simulink model "mathmeticmodel"  (R2019b)
settings: Solver=VariableStepAuto  StartTime=0.0  StopTime=10  RelTol=1e-3
undefined symbols (not defined in the file): DiscIntNeverNeededParam, eta, Fh, Id0, k, KL, KR, LdRated, LqRated, psi_dh, psi_qh, PsiPMRated, RsRated, TsimFSO, TsimMotor, Ud0, Udh, Uq0, Uqh, we
libraries: simulink x2
settings Model: SimulationMode=accelerator  Creator=Downstream  LastModifiedBy=Downstream
settings DataIOCC: ReturnWorkspaceOutputs=off

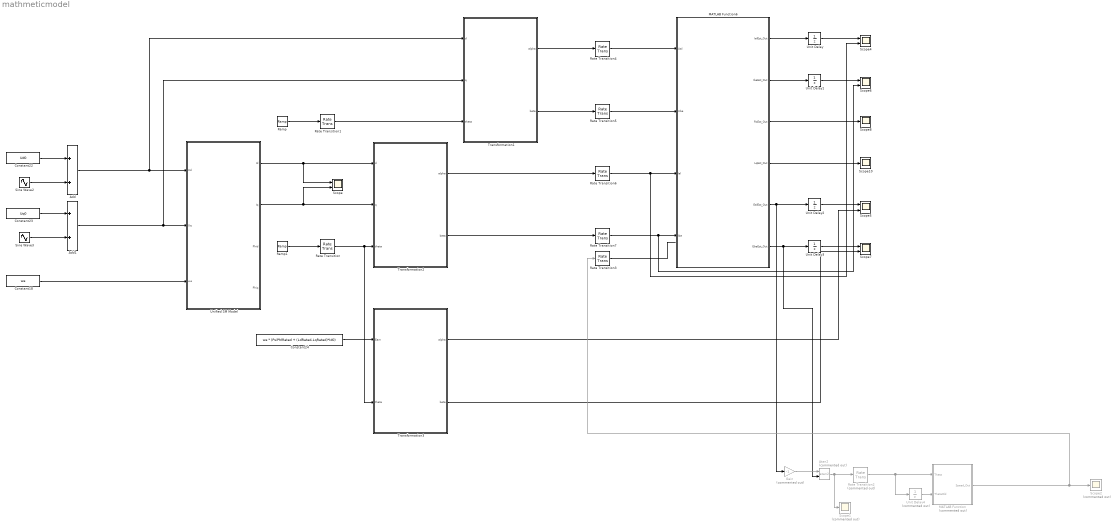
== system mathmeticmodel ==
  Add : Sum
  Add1 : Sum
  Atan2 : Trigonometry  Commented=on  Operator=atan2
  Constant18 : Constant  Value=we  SampleTime=TsimFSO
  Constant22 : Constant  Value=Ud0  SampleTime=TsimFSO
  Constant23 : Constant  Value=Uq0  SampleTime=TsimFSO
  Constant24 : Constant  Value=we * (PsiPMRated + (LdRated-LqRated)*Id0)  SampleTime=TsimMotor
  Gain : Gain  Commented=on  Gain=-1
  MATLAB Function : MATLAB Function  Commented=on  TreatAsAtomicUnit=on
  MATLAB Function6 : MATLAB Function  TreatAsAtomicUnit=on
  Ramp : simulink/Sources/Ramp  slope=we  start=0  InitialOutput=0
  Ramp1 : simulink/Sources/Ramp  slope=we  start=0  InitialOutput=0
  Rate Transition : RateTransition  OutPortSampleTime=TsimMotor
  Rate Transition1 : RateTransition  OutPortSampleTime=TsimMotor
  Rate Transition2 : RateTransition  Commented=on  OutPortSampleTime=TsimFSO*10
  Rate Transition{3..7} (5 alike) : RateTransition  OutPortSampleTime=TsimFSO
  Scope{,4..7} (5 alike) : Scope  NumInputPorts=2
  Scope1 : Scope  Commented=on
  Scope10 : Scope
  Scope2 : Scope  Commented=on
  Scope8 : Scope
  Sine Wave2 : Sin  Amplitude=Udh  Frequency=Fh * 2 * pi  Phase=psi_dh  SampleTime=TsimFSO
  Sine Wave3 : Sin  Amplitude=Uqh  Frequency=Fh * 2 * pi  Phase=psi_qh  SampleTime=TsimFSO
  Transformation1 : Subsystem
  Transformation2 : Subsystem
  Transformation3 : Subsystem
  Unified SM Model : Subsystem
  Unit Delay : UnitDelay  SampleTime=-1  HasFrameUpgradeWarning=on
  Unit Delay1 : UnitDelay  SampleTime=-1  HasFrameUpgradeWarning=on
  Unit Delay2 : UnitDelay  SampleTime=TsimFSO  HasFrameUpgradeWarning=on
  Unit Delay3 : UnitDelay  SampleTime=TsimFSO  HasFrameUpgradeWarning=on
  Unit Delay4 : UnitDelay  Commented=on  SampleTime=-1  HasFrameUpgradeWarning=on
  wires:
  Constant22/1 -> Add/1
  Constant23/1 -> Add1/1
  Sine Wave2/1 -> Add/2
  Sine Wave3/1 -> Add1/2
  Unified SM Model/1(Id) -> Scope/1, Transformation2/1(d)
  Unified SM Model/2(Iq) -> Scope/2, Transformation2/2(q)
  Constant18/1 -> Unified SM Model/3(we)
  Ramp1/1 -> Rate Transition/1
  Rate Transition/1 -> Transformation2/3(theta), Transformation3/2(theta)
  Rate Transition1/1 -> Transformation1/3(theta)
  Ramp/1 -> Rate Transition1/1
  Transformation1/1(alpha) -> Rate Transition4/1
  Transformation1/2(beta) -> Rate Transition5/1
  Transformation2/1(alpha) -> Rate Transition6/1
  Transformation2/2(beta) -> Rate Transition7/1
  MATLAB Function6/1(IalEst_Out) -> Unit Delay/1
  MATLAB Function6/5(EalEst_Out) -> Unit Delay2/1, Gain/1
  MATLAB Function6/2(IbeEst_Out) -> Unit Delay1/1
  Constant24/1 -> Transformation3/1(Eam)
  MATLAB Function6/3(RsEst_Out) -> Scope8/1
  MATLAB Function6/4(LqEst_Out) -> Scope10/1
  Rate Transition6/1 -> MATLAB Function6/3(Ial), Scope4/2
  Rate Transition7/1 -> MATLAB Function6/4(Ibe), Scope6/2
  Unit Delay/1 -> Scope4/1
  Unit Delay1/1 -> Scope6/1
  Transformation3/1(alpha) -> Scope5/2
  Transformation3/2(beta) -> Scope7/2
  Unit Delay2/1 -> Scope5/1
  Unit Delay3/1 -> Scope7/1
  Add/1 -> Transformation1/1(d), Unified SM Model/1(Ud)
  Add1/1 -> Transformation1/2(q), Unified SM Model/2(Uq)
  Rate Transition4/1 -> MATLAB Function6/1(Ual)
  Rate Transition5/1 -> MATLAB Function6/2(Ube)
  MATLAB Function6/6(EbeEst_Out) -> Atan2/2, Unit Delay3/1
  Gain/1 -> Atan2/1
  Atan2/1 -> Rate Transition2/1, Scope1/1
  Unit Delay4/1 -> MATLAB Function/2(ThetaOld)
  Rate Transition2/1 -> Unit Delay4/1, MATLAB Function/1(Theta)
  Rate Transition3/1 -> ?
  MATLAB Function/1(Speed_Out) -> Rate Transition3/1, Scope2/1

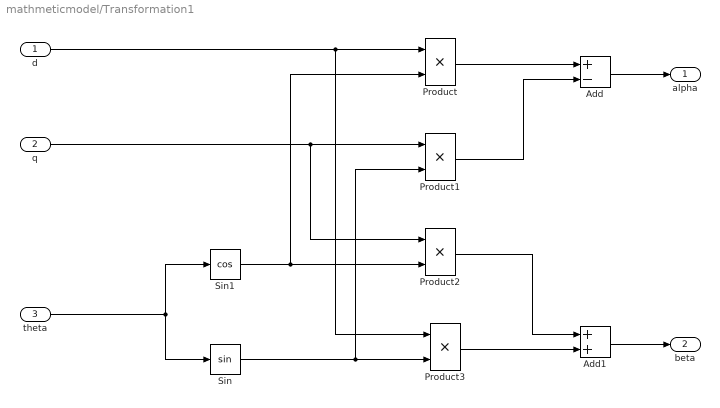
== system mathmeticmodel/Transformation1 ==
  d : Inport
  q : Inport  Port=2
  theta : Inport  Port=3
  Add : Sum  Inputs=+-
  Add1 : Sum
  Product{,1..3} (4 alike) : Product
  Sin : Trigonometry  OutputSignalType=real
  Sin1 : Trigonometry  Operator=cos  OutputSignalType=real
  alpha : Outport
  beta : Outport  Port=2
  wires:
  Product/1 -> Add/1
  Sin/1 -> Product3/2, Product1/2
  Product1/1 -> Add/2
  Add1/1 -> beta/1
  Sin1/1 -> Product2/2, Product/2
  Product2/1 -> Add1/1
  d/1 -> Product3/1, Product/1
  q/1 -> Product2/1, Product1/1
  Product3/1 -> Add1/2
  Add/1 -> alpha/1
  theta/1 -> Sin/1, Sin1/1

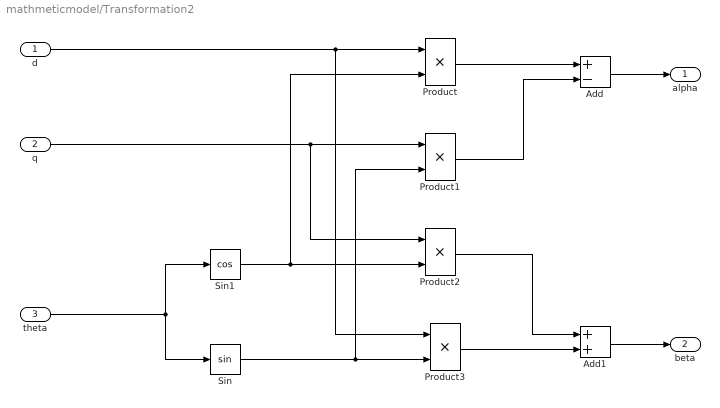
== system mathmeticmodel/Transformation2 ==
  d : Inport
  q : Inport  Port=2
  theta : Inport  Port=3
  Add : Sum  Inputs=+-
  Add1 : Sum
  Product{,1..3} (4 alike) : Product
  Sin : Trigonometry  OutputSignalType=real
  Sin1 : Trigonometry  Operator=cos  OutputSignalType=real
  alpha : Outport
  beta : Outport  Port=2
  wires:
  Product/1 -> Add/1
  Sin/1 -> Product3/2, Product1/2
  Product1/1 -> Add/2
  Add1/1 -> beta/1
  Sin1/1 -> Product2/2, Product/2
  Product2/1 -> Add1/1
  d/1 -> Product3/1, Product/1
  q/1 -> Product2/1, Product1/1
  Product3/1 -> Add1/2
  Add/1 -> alpha/1
  theta/1 -> Sin/1, Sin1/1

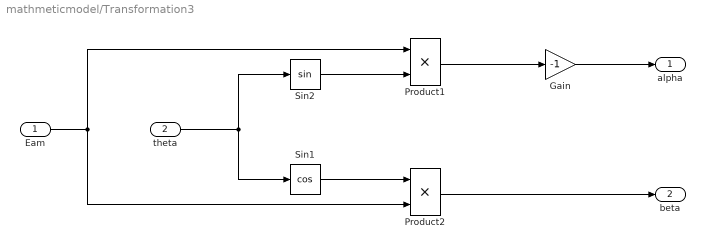
== system mathmeticmodel/Transformation3 ==
  Eam : Inport
  theta : Inport  Port=2
  Gain : Gain  Gain=-1
  Product1 : Product
  Product2 : Product
  Sin1 : Trigonometry  Operator=cos  OutputSignalType=real
  Sin2 : Trigonometry  OutputSignalType=real
  alpha : Outport
  beta : Outport  Port=2
  wires:
  theta/1 -> Sin2/1, Sin1/1
  Product1/1 -> Gain/1
  Product2/1 -> beta/1
  Eam/1 -> Product1/1, Product2/2
  Sin2/1 -> Product1/2
  Gain/1 -> alpha/1
  Sin1/1 -> Product2/1

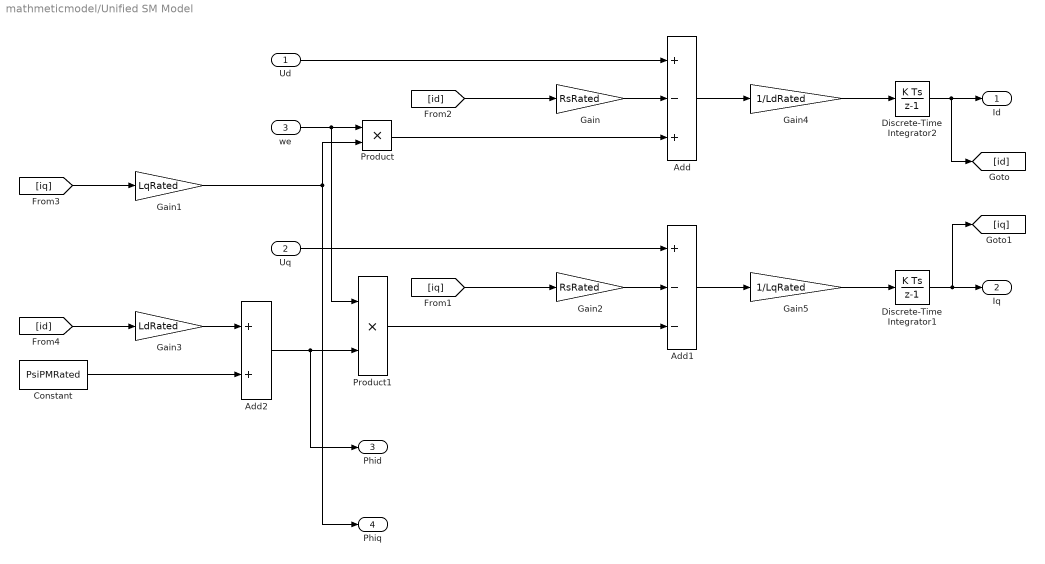
== system mathmeticmodel/Unified SM Model ==
  Ud : Inport
  Uq : Inport  Port=2
  we : Inport  Port=3
  Add : Sum  Inputs=+-+
  Add1 : Sum  Inputs=+--
  Add2 : Sum
  Constant : Constant  Value=PsiPMRated  SampleTime=TsimMotor
  Discrete-Time Integrator1 : DiscreteIntegrator  SampleTime=TsimMotor  UpperSaturationLimit=0  LowerSaturationLimit=-400  ICPrevOutput=DiscIntNeverNeededParam  ICPrevScaledInput=DiscIntNeverNeededParam
  Discrete-Time Integrator2 : DiscreteIntegrator  SampleTime=TsimMotor  UpperSaturationLimit=0  LowerSaturationLimit=-400  ICPrevOutput=DiscIntNeverNeededParam  ICPrevScaledInput=DiscIntNeverNeededParam
  Gain : Gain  Gain=RsRated
  Gain1 : Gain  Gain=LqRated
  Gain2 : Gain  Gain=RsRated
  Gain3 : Gain  Gain=LdRated
  Gain4 : Gain  Gain=1/LdRated
  Gain5 : Gain  Gain=1/LqRated
  Product : Product
  Product1 : Product
  Id : Outport
  Iq : Outport  Port=2
  Phid : Outport  Port=3
  Phiq : Outport  Port=4
  wires:
  Ud/1 -> Add/1
  we/1 -> Product/1, Product1/1
  Gain/1 -> Add/2
  [iq] -> Gain1/1
  [id] -> Gain/1
  Add/1 -> Gain4/1
  [id] -> Gain3/1
  [iq] -> Gain2/1
  Gain2/1 -> Add1/2
  Uq/1 -> Add1/1
  Gain3/1 -> Add2/1
  Constant/1 -> Add2/2
  Add2/1 -> Phid/1, Product1/2
  Product1/1 -> Add1/3
  Add1/1 -> Gain5/1
  Gain4/1 -> Discrete-Time Integrator2/1
  Gain5/1 -> Discrete-Time Integrator1/1
  Discrete-Time Integrator2/1 -> [id], Id/1
  Discrete-Time Integrator1/1 -> [iq], Iq/1
  Gain1/1 -> Phiq/1, Product/2
  Product/1 -> Add/3

== matlab function mathmeticmodel/MATLAB Function ==
  data: Theta input; Speed_Out output; ThetaOld input
function Speed_Out = fcn(Theta,ThetaOld)
persistent Speed
if isempty(Speed)
    Speed = 250;
end
Temp = (Theta - ThetaOld);
if(Temp < -pi)
    Temp = Temp + 2 * pi;
end
Speed_new = Temp/(1e-3);
Speed = Speed * 0.999 + Speed_new * 0.001;
Speed_Out = Speed;

== matlab function mathmeticmodel/MATLAB Function6 ==
  data: Ual input; IalEst_Out output; Ube input; Ial input; Ibe input; k parameter; IbeEst_Out output; RsEst_Out output; LqEst_Out output; RsRated parameter; LqRated parameter; EalEst_Out output; EbeEst_Out output; eta parameter; TsimFSO parameter; PsiPMRated parameter; KL parameter; KR parameter; we parameter
function [IalEst_Out,IbeEst_Out,RsEst_Out,LqEst_Out,EalEst_Out,EbeEst_Out] = FSO(Ual,Ube,Ial,Ibe,k,RsRated, LqRated, eta,TsimFSO,PsiPMRated,KL, KR, we)
persistent IalEst IbeEst RsEst LqEst EalEst EbeEst;
if isempty(IalEst)
    IalEst = 0;
    IbeEst = 0;
    EalEst = 0;
    EbeEst = 0 * PsiPMRated;
    RsEst = RsRated;
    LqEst = LqRated;
end
Ts = TsimFSO;
AI = [-RsEst/LqEst 0;0 -RsEst/LqEst];
BI = [1/LqEst 0; 0 1/LqEst];
PhiII = eye(2) + Ts * AI + 1/2 * Ts^2 * AI^2;
GIU   = (Ts * eye(2) + 0.5 * Ts^2 * AI + 1/6 * Ts^3 * AI^2) * BI;
% GIU   = (Ts * eye(2) + Ts^2 * AI + 1/2 * Ts^3 * AI^2) * BI;
% PhiII = eye(2) + Ts * AI;
% GIU   = (Ts * eye(2)) * BI;
GIE   = -GIU;
GIK   = GIU * k;
Xk_hat = [IalEst,IbeEst]';Uk = [Ual,Ube]';Ek_hat=[EalEst,EbeEst]';Xk = [Ial,Ibe]';
X_tilde = Xk_hat - Xk;
sgn = sign(X_tilde);
Xk_pre = PhiII * Xk_hat + GIE * Ek_hat + GIU * Uk + GIK * sgn;
dot_i_hat = (1/LqEst)*(Uk - RsEst * Xk_hat - Ek_hat);
Rs_hat_dot = KR * (X_tilde') * (Xk_hat);
Lq_hat_dot = KL * (X_tilde') * (dot_i_hat);


IalEst = Xk_pre(1);IbeEst = Xk_pre(2);
IalEst_Out = IalEst; IbeEst_Out = IbeEst;

T = k*[eta,we;-we,eta];
AE = [0 -we;we 0];
PhiEE = eye(2) + Ts * AE + 1/2 * Ts^2 * AE^2;
GET   = (Ts * eye(2) + 0.5 * Ts^2 * AE + 1/6 * Ts^3 * AE^2) * T;
% GET   = (Ts * eye(2) + Ts^2 * AE) * T;
% PhiEE = eye(2) + Ts * AE;
% GET   = (Ts * eye(2)) * T;
Ekp_pre= PhiEE * Ek_hat + GET * sgn;
EalEst = Ekp_pre(1);EbeEst = Ekp_pre(2);
EalEst_Out = EalEst; EbeEst_Out = EbeEst;

RsEst_Out = RsEst + Rs_hat_dot * Ts + 0.5 * Rs_hat_dot^2 * Ts^2;
LqEst_Out = LqEst + Lq_hat_dot * Ts + 0.5 * Lq_hat_dot^2 * Ts^2;
if(RsEst_Out > RsRated * 2)
    RsEst_Out = RsRated * 2;
elseif(RsEst_Out < RsRated / 2)
    RsEst_Out = RsRated / 2;
end

if(LqEst_Out > LqRated * 2)
    LqEst_Out = LqRated * 2;
elseif(LqEst_Out < LqRated / 2)
    LqEst_Out = LqRated / 2;
end
    
RsEst = RsEst_Out;
LqEst = LqEst_Out;
end
